simulink model "CB_core_control"  (R2023b)
settings: configuration reference "slow_tsk_conf" (kept outside this file)
undefined symbols (not defined in the file): slow_tsk_st
libraries: eeGeneralControl x1
settings Model: DataDictionary=fmuGenerationDictionay.sldd  ModifiedByFormat=Third Equation Ltd  Creator=Third Equation Ltd  LastModifiedBy=Third Equation Ltd
settings ConfigSetRef: SourceName=slow_tsk_conf

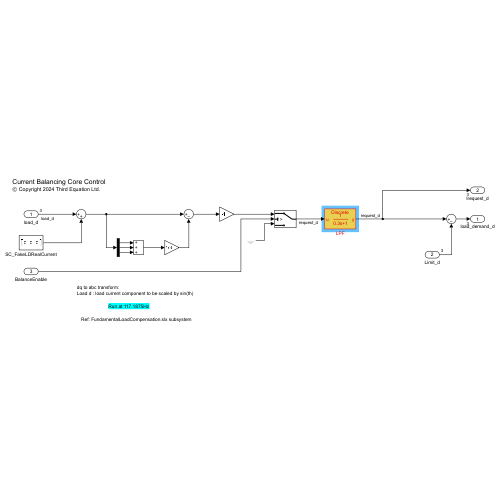
[thumbnail: Simulink's stored preview of the top-level diagram]
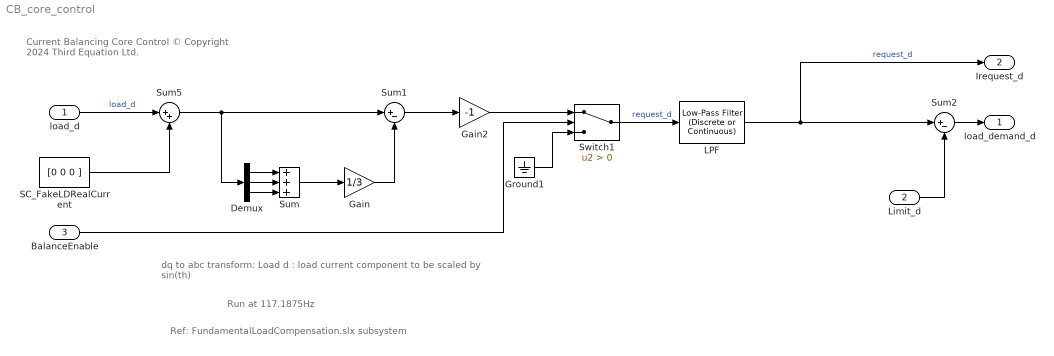
== system CB_core_control ==
  note: Ref: FundamentalLoadCompensation.slx subsystem
  note: dq to abc transform:
      | Load d : load current component to be scaled by sin(th)
  note: Current Balancing Core Control
      | © Copyright 2024 Third Equation Ltd.
  note: Run at 117.1875Hz
  load_d : Inport  OutDataTypeStr=single  PortDimensions=3
  Limit_d : Inport  Port=2  OutDataTypeStr=single  PortDimensions=3
  BalanceEnable : Inport  Port=3  OutDataTypeStr=boolean  PortDimensions=1
  Demux : Demux  Outputs=3
  Gain : Gain  Gain=1/3
  Gain2 : Gain  Gain=-1
  Ground1 : Ground
  LPF : eeGeneralControl/Low-Pass Filter (Discrete or Continuous)  K=1  T=0.3  B=inf  A=-inf  init_option=Inherited from block input  x0=0  Ts=slow_tsk_st
  SC_FakeLDRealCurrent : Constant  Value=[0 0 0 ]  OutDataTypeStr=single
  Sum : Sum  Inputs=+++
  Sum1 : Sum  Inputs=|+-
  Sum2 : Sum  Inputs=|+-
  Sum5 : Sum  Inputs=|++
  Switch1 : Switch  Criteria=u2 > Threshold  SaturateOnIntegerOverflow=off  InputSameDT=off
  load_demand_d : Outport  OutDataTypeStr=single  PortDimensions=3
  Irequest_d : Outport  Port=2  OutDataTypeStr=single  PortDimensions=3
  wires:
  LPF/1 -> Sum2/1, Irequest_d/1  "request_d"
  Sum/1 -> Gain/1
  Switch1/1 -> LPF/1  "request_d"
  SC_FakeLDRealCurrent/1 -> Sum5/2
  load_d/1 -> Sum5/1  "load_d"
  Sum1/1 -> Gain2/1
  Gain2/1 -> Switch1/1
  BalanceEnable/1 -> Switch1/2
  Sum2/1 -> load_demand_d/1
  Limit_d/1 -> Sum2/2
  Sum5/1 -> Demux/1, Sum1/1
  Demux/1 -> Sum/1
  Ground1/1 -> Switch1/3
  Demux/2 -> Sum/2
  Gain/1 -> Sum1/2
  Demux/3 -> Sum/3
